simulink model "LAB1_5_sim"  (R2025b)
settings: Solver=VariableStepAuto  StartTime=0.0  StopTime=5  RelTol=1e-3
undefined symbols (not defined in the file or in its folder): A_a, B_a, Beq, C_p, daq, drv, gbox, Jeq, K, mot, pulse2deg, rads2rpm, Req, w0
settings Model: Creator=Gioele  LastModifiedBy=Gioele

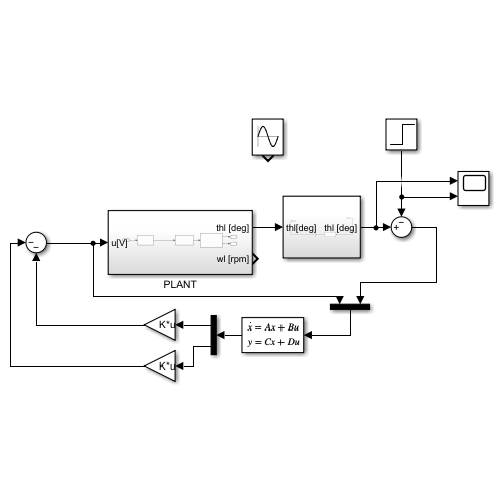
[thumbnail: Simulink's stored preview of the top-level diagram]
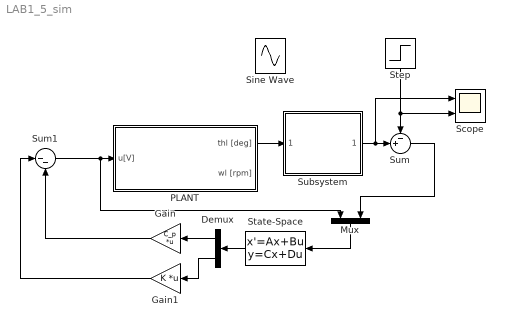
== system LAB1_5_sim ==
  Demux : Demux  Outputs=2
  Gain : Gain  Gain=C_p  Multiplication=Matrix(K*u)
  Gain1 : Gain  Gain=K  Multiplication=Matrix(K*u)
  Mux : Mux  Inputs=2
  PLANT : Subsystem
  Scope : Scope  NumInputPorts=2
      settings: ActiveDisplayYMinimum=-54.449999999999996  ActiveDisplayYMaximum=56.25
  Sine Wave : Sin  Amplitude=30  Frequency=w0  SampleTime=0
  State-Space : StateSpace  A=A_a  B=B_a  C=eye(5)  D=[0 0;0 0;0 0;0 0;0 0]  InitialCondition=0
  Step : Step  Time=0  After=70  SampleTime=0
  Subsystem : Subsystem
  Sum : Sum  Inputs=-+|
  Sum1 : Sum  Inputs=|--
  wires:
  Step/1 -> Scope/2, Sum/1
  PLANT/1(thl [deg]) -> Subsystem/1(thl[deg])
  Subsystem/1(thl [deg]) -> Scope/1, Sum/2
  State-Space/1 -> Demux/1
  Demux/1 -> Gain/1
  Demux/2 -> Gain1/1
  Gain/1 -> Sum1/2
  Gain1/1 -> Sum1/1
  Sum1/1 -> Mux/1, PLANT/1(u[V])
  Sum/1 -> Mux/2
  Mux/1 -> State-Space/1

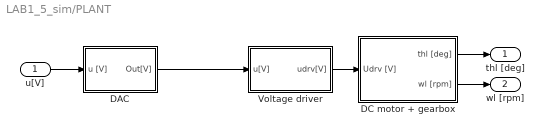
== system LAB1_5_sim/PLANT ==
  u[V] : Inport
  DAC : Subsystem  TreatAsAtomicUnit=on
  DC motor + gearbox : Subsystem
  Voltage driver : Subsystem  TreatAsAtomicUnit=on
  thl [deg] : Outport
  wl [rpm] : Outport  Port=2
  wires:
  Voltage driver/1(udrv[V]) -> DC motor + gearbox/1(Udrv [V])
  DC motor + gearbox/2(wl [rpm]) -> wl [rpm]/1
  DC motor + gearbox/1(thl [deg]) -> thl [deg]/1
  u[V]/1 -> DAC/1(u [V])
  DAC/1(Out[V]) -> Voltage driver/1(u[V])

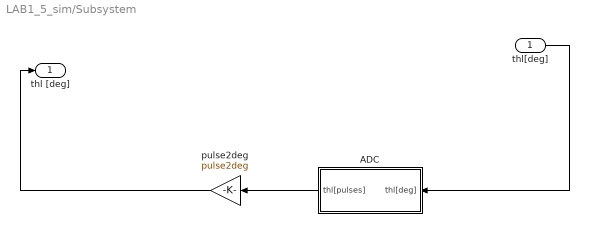
== system LAB1_5_sim/Subsystem ==
  thl[deg] : Inport
  ADC : Subsystem  TreatAsAtomicUnit=on
  pulse2deg : Gain  Gain=pulse2deg
  thl [deg] : Outport
  wires:
  ADC/1(thl[pulses]) -> pulse2deg/1
  thl[deg]/1 -> ADC/1(thl[deg])
  pulse2deg/1 -> thl [deg]/1

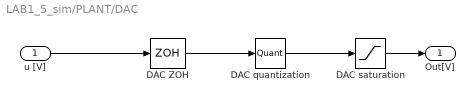
== system LAB1_5_sim/PLANT/DAC ==
  u [V] : Inport
  "DAC ZOH " : ZeroOrderHold  SampleTime=daq.dac.Ts
  DAC quantization : Quantizer  QuantizationInterval=daq.dac.q
  DAC saturation : Saturate  UpperLimit=daq.dac.fs  LowerLimit=-daq.dac.fs
  Out[V] : Outport
  wires:
  DAC quantization/1 -> DAC saturation/1
  u [V]/1 -> "DAC ZOH "/1
  "DAC ZOH "/1 -> DAC quantization/1
  DAC saturation/1 -> Out[V]/1

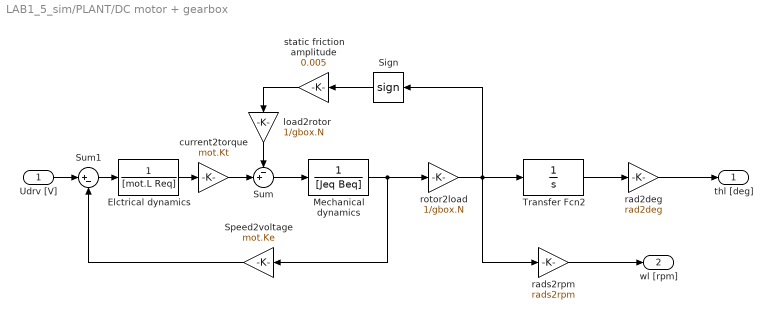
== system LAB1_5_sim/PLANT/DC motor + gearbox ==
  Udrv [V] : Inport
  Elctrical dynamics : TransferFcn  Denominator=[mot.L Req]
  Mechanical dynamics : TransferFcn  Denominator=[Jeq Beq]
  Sign : Signum  ZeroCross=off
  Speed2voltage : Gain  Gain=mot.Ke
  Sum : Sum  Inputs=-+|
  Sum1 : Sum  Inputs=|+-
  Transfer Fcn2 : TransferFcn  Denominator=[1 0]
  current2torque : Gain  Gain=mot.Kt
  load2rotor : Gain  Gain=1/gbox.N
  rad2deg : Gain  Gain=rad2deg
  rads2rpm : Gain  Gain=rads2rpm
  rotor2load : Gain  Gain=1/gbox.N
  static friction amplitude : Gain  Gain=0.005
  thl [deg] : Outport
  wl [rpm] : Outport  Port=2
  wires:
  rotor2load/1 -> Sign/1, rads2rpm/1, Transfer Fcn2/1
  Sign/1 -> static friction amplitude/1
  rads2rpm/1 -> wl [rpm]/1
  Sum/1 -> Mechanical dynamics/1
  Udrv [V]/1 -> Sum1/1
  static friction amplitude/1 -> load2rotor/1
  load2rotor/1 -> Sum/1
  Transfer Fcn2/1 -> rad2deg/1
  current2torque/1 -> Sum/2
  Speed2voltage/1 -> Sum1/2
  Mechanical dynamics/1 -> Speed2voltage/1, rotor2load/1
  Elctrical dynamics/1 -> current2torque/1
  Sum1/1 -> Elctrical dynamics/1
  rad2deg/1 -> thl [deg]/1

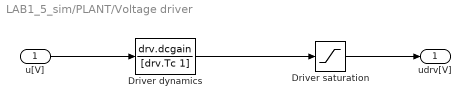
== system LAB1_5_sim/PLANT/Voltage driver ==
  u[V] : Inport  OutMax=[5]
  Driver dynamics : TransferFcn  Numerator=drv.dcgain  Denominator=[drv.Tc 1]
  Driver saturation : Saturate  UpperLimit=drv.outmax  LowerLimit=-drv.outmax
  udrv[V] : Outport
  wires:
  Driver dynamics/1 -> Driver saturation/1
  u[V]/1 -> Driver dynamics/1
  Driver saturation/1 -> udrv[V]/1

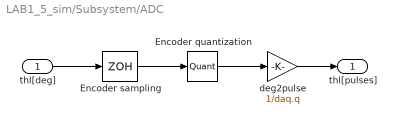
== system LAB1_5_sim/Subsystem/ADC ==
  thl[deg] : Inport
  Encoder quantization : Quantizer  QuantizationInterval=daq.q
  Encoder sampling : ZeroOrderHold  SampleTime=daq.dac.Ts
  deg2pulse : Gain  Gain=1/daq.q
  thl[pulses] : Outport
  wires:
  Encoder quantization/1 -> deg2pulse/1
  thl[deg]/1 -> Encoder sampling/1
  Encoder sampling/1 -> Encoder quantization/1
  deg2pulse/1 -> thl[pulses]/1
